simulink model "img"  (R2016a)
settings: Solver=VariableStepAuto  StartTime=0.0  StopTime=1  RelTol=1e-3
undefined symbols (not defined in the file or in its folder): gray
libraries: visionanalysis x4, visionsources x4, fuzblock x1
settings Model: Creator=Shadhin  LastModifiedBy=Shadhin

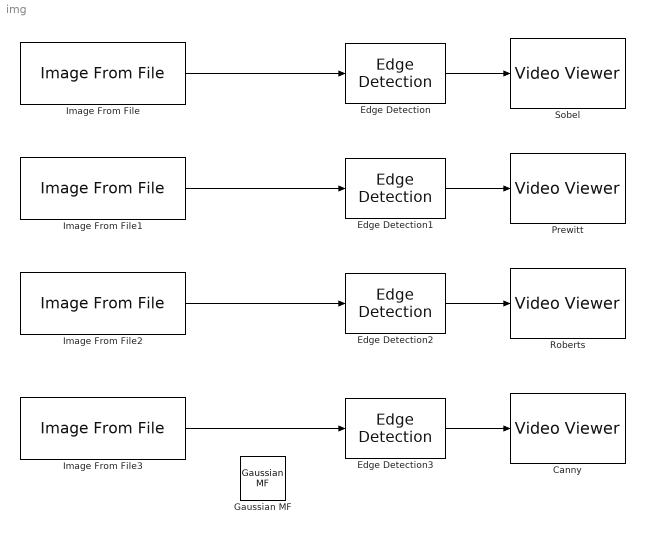
== system img ==
  Canny : VideoViewer  colormapValue=gray(256)  FigPos=[670 627 571 362]
  Edge Detection : visionanalysis/Edge Detection  method=Sobel  outputType=Binary image  userDefinedThreshold=off  thresholdSource=Input port  threshold=20  thresholdTuning=4  edgeThinning=off  threshold_canny=[0.25 0.60]  autoPercent=70  sigma=1  prodOutputMode=Binary point scaling  prodOutputWordLength=32  prodOutputFracLength=8  roundingMode=Round  overflowMode=off
  Edge Detection1 : visionanalysis/Edge Detection  method=Prewitt  outputType=Binary image  userDefinedThreshold=off  thresholdSource=Input port  threshold=20  thresholdTuning=4  edgeThinning=off  threshold_canny=[0.25 0.60]  autoPercent=70  sigma=1  prodOutputMode=Binary point scaling  prodOutputWordLength=32  prodOutputFracLength=8  roundingMode=Round  overflowMode=off
  Edge Detection2 : visionanalysis/Edge Detection  method=Roberts  outputType=Binary image  userDefinedThreshold=off  thresholdSource=Input port  threshold=20  thresholdTuning=4  edgeThinning=off  threshold_canny=[0.25 0.60]  autoPercent=70  sigma=1  prodOutputMode=Binary point scaling  prodOutputWordLength=32  prodOutputFracLength=8  roundingMode=Round  overflowMode=off
  Edge Detection3 : visionanalysis/Edge Detection  method=Canny  outputType=Binary image  userDefinedThreshold=off  thresholdSource=Input port  threshold=20  thresholdTuning=4  edgeThinning=off  threshold_canny=[0.25 0.60]  autoPercent=70  sigma=1  prodOutputMode=Binary point scaling  prodOutputWordLength=32  prodOutputFracLength=8  roundingMode=Round  overflowMode=off
  Gaussian MF : fuzblock/Membership  Functions/Gaussian MF  sigma=1  mu=0
  Image From File : visionsources/Image From File  Tag=vipblks_nd  FileName=C:\Program Files\MATLAB\R2016a\toolbox\images\imdata\coins.png  imagePorts=One multidimensional signal  Ts=1  ImageDataType=uint8  Signed=on  WordLength=16  sdImageDataType=uint(8)  FractionLengthMode=User-defined  FractionLength=15  OutPortLabels=R|G|B
  Image From File1 : visionsources/Image From File  Tag=vipblks_nd  FileName=C:\Program Files\MATLAB\R2016a\toolbox\images\imdata\blobs.png  imagePorts=One multidimensional signal  Ts=2  ImageDataType=uint8  Signed=on  WordLength=16  sdImageDataType=uint(8)  FractionLengthMode=User-defined  FractionLength=15  OutPortLabels=R|G|B
  Image From File2 : visionsources/Image From File  Tag=vipblks_nd  FileName=C:\Program Files\MATLAB\R2016a\toolbox\images\imdata\blobs.png  imagePorts=One multidimensional signal  Ts=3  ImageDataType=uint8  Signed=on  WordLength=16  sdImageDataType=uint(8)  FractionLengthMode=User-defined  FractionLength=15  OutPortLabels=R|G|B
  Image From File3 : visionsources/Image From File  Tag=vipblks_nd  FileName=C:\Program Files\MATLAB\R2016a\toolbox\images\imdata\blobs.png  imagePorts=One multidimensional signal  Ts=4  ImageDataType=double  Signed=on  WordLength=16  sdImageDataType=uint(8)  FractionLengthMode=User-defined  FractionLength=15  OutPortLabels=R|G|B
  "Prewitt " : VideoViewer  colormapValue=gray(256)  FigPos=[614 668 571 362]
  Roberts : VideoViewer  colormapValue=gray(256)  FigPos=[146 677 571 362]
  "Sobel " : VideoViewer  colormapValue=gray(256)  FigPos=[204 682 571 362]
  wires:
  Image From File/1 -> Edge Detection/1
  Edge Detection/1 -> "Sobel "/1
  Image From File1/1 -> Edge Detection1/1
  Edge Detection1/1 -> "Prewitt "/1
  Image From File2/1 -> Edge Detection2/1
  Edge Detection2/1 -> Roberts/1
  Edge Detection3/1 -> Canny/1
  Image From File3/1 -> Edge Detection3/1
